simulink model "Arduino_Test"  (R2020b)
settings: Solver=VariableStepAuto  StartTime=0.0  StopTime=10.0  RelTol=1e-3
libraries: arduinolib x1
settings Model: Creator=Student  LastModifiedBy=Student

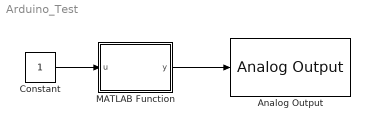
== system Arduino_Test ==
  Analog Output : arduinolib/Analog Output  DACpin=DAC0  blockPlatform=arduino
      settings: SourceProductBaseCode=ARDUINO
  Constant : Constant
  MATLAB Function : MATLAB Function  TreatAsAtomicUnit=on
  wires:
  MATLAB Function/1(y) -> Analog Output/1
  Constant/1 -> MATLAB Function/1(u)

== matlab function Arduino_Test/MATLAB Function ==
  data: u input; y output
function y = fcn(u)

y = typecast(4098 * u,'uint16');
